simulink model "Disturbance_observer"  (R2012b)
settings: Solver=ode3  StartTime=0.0  StopTime=20  FixedStep=0.001  RelTol=1e-3
libraries: simulink x3
settings Model: Creator=mchusr  LastModifiedBy=mchusr

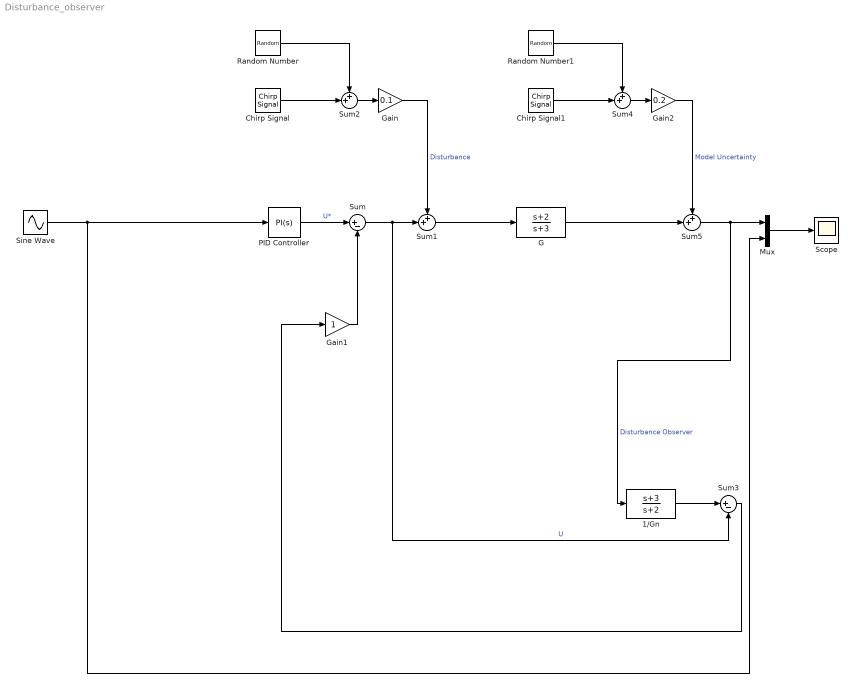
== system Disturbance_observer ==
  1/Gn : TransferFcn  Numerator=[1 3]  Denominator=[1 2]
  Chirp Signal : simulink/Sources/Chirp Signal  f1=0.04  T=30  f2=0.3
  Chirp Signal1 : simulink/Sources/Chirp Signal  f1=0.04  T=30  f2=0.3
  G : TransferFcn  Numerator=[1 2]  Denominator=[1 3]
  Gain : Gain  Gain=0.1
  Gain1 : Gain
  Gain2 : Gain  Gain=0.2
  Mux : Mux  Inputs=2
  PID Controller : simulink/Continuous/PID Controller  Controller=PI  TimeDomain=Continuous-time  SampleTime=1  IntegratorMethod=Forward Euler  FilterMethod=Forward Euler  Form=Parallel  P=1.5  I=0.02  D=0.3  N=100  InitialConditionSource=internal  InitialConditionForIntegrator=0  InitialConditionForFilter=0  ExternalReset=none  LimitOutput=off  UpperSaturationLimit=inf  LowerSaturationLimit=-inf  LinearizeAsGain=on  AntiWindupMode=none  Kb=1  TrackingMode=off  Kt=1  PParamMin=[]  PParamMax=[]  IParamMin=[]  IParamMax=[]  DParamMin=[]  DParamMax=[]  NParamMin=[]  NParamMax=[]  KbParamMin=[]  KbParamMax=[]  KtParamMin=[]  KtParamMax=[]  POutMin=[]  POutMax=[]  IOutMin=[]  IOutMax=[]  DOutMin=[]  DOutMax=[]  NOutMin=[]  NOutMax=[]  KbOutMin=[]  KbOutMax=[]  KtOutMin=[]  KtOutMax=[]  IntegratorOutMin=[]  IntegratorOutMax=[]  FilterOutMin=[]  FilterOutMax=[]  SumOutMin=[]  SumOutMax=[]  SumI1OutMin=[]  SumI1OutMax=[]  SumI2OutMin=[]  SumI2OutMax=[]  SumI3OutMin=[]  SumI3OutMax=[]  SumDOutMin=[]  SumDOutMax=[]  SaturationOutMin=[]  SaturationOutMax=[]  IntegratorContinuousStateAttributes=''  IntegratorStateMustResolveToSignalObject=off  IntegratorRTWStateStorageClass=Auto  FilterContinuousStateAttributes=''  FilterStateMustResolveToSignalObject=off  FilterRTWStateStorageClass=Auto
  Random Number : RandomNumber  SampleTime=0.001
  Random Number1 : RandomNumber  SampleTime=0.001
  Scope : Scope
      settings: TimeRange=10  YMin=0  YMax=1
  Sine Wave : Sin  SampleTime=0
  Sum : Sum  Inputs=|+-
  Sum{1..2,4..5} (4 alike) : Sum  Inputs=++|
  Sum3 : Sum  Inputs=|+-
  wires:
  PID Controller/1 -> Sum/1  "U*"
  Sum1/1 -> G/1
  Chirp Signal/1 -> Sum2/2
  Gain/1 -> Sum1/1  "Disturbance"
  Sum2/1 -> Gain/1
  Random Number/1 -> Sum2/1
  Mux/1 -> Scope/1
  Sine Wave/1 -> PID Controller/1, Mux/2
  G/1 -> Sum5/2
  1/Gn/1 -> Sum3/1
  Sum3/1 -> Gain1/1
  Sum/1 -> Sum3/2, Sum1/2  "U"
  Gain1/1 -> Sum/2
  Chirp Signal1/1 -> Sum4/2
  Gain2/1 -> Sum5/1  "Model Uncertainty"
  Sum4/1 -> Gain2/1
  Random Number1/1 -> Sum4/1
  Sum5/1 -> 1/Gn/1, Mux/1  "Disturbance Observer"
